simulink model "lab131"  (R2015b)
settings: Solver=ode15s  SolverMode=SingleTasking  StartTime=0.0  StopTime=0.01  RelTol=1e-3
libraries: fl_lib x8, nesl_utility x5, simulink x1
settings Model: Creator=Peter  LastModifiedBy=Peter
settings DataIOCC: LimitDataPoints=off
settings DebuggingCC: AllowSymbolicDim=on  SFUnexpectedBacktrackingDiag=error  SFNoUnconditionalDefaultTransitionDiag=error
settings ModelReferenceCC: PropagateSignalLabelsOutOfModel=on
settings GRTTargetCC: TargetLangStandard=C99 (ISO)
settings ConfigComp: CovMetricSettings=dwe  CovHtmlReporting=off  CovSaveCumulativeToWorkspaceVar=off  CovSaveSingleToWorkspaceVar=off  CovModelRefEnable=Off  CovExternalEMLEnable=on
settings ConfigurationSet: Description=Simscape Multibody

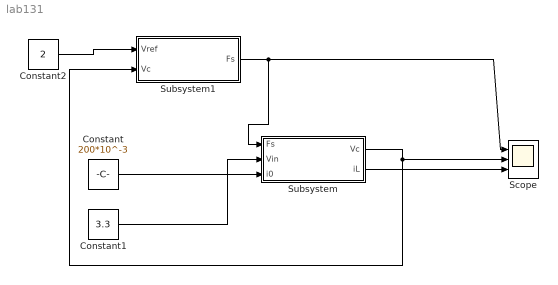
== system lab131 ==
  Constant : Constant  Value=200*10^-3
  Constant1 : Constant  Value=3.3
  Constant2 : Constant  Value=2
  Scope : Scope  NumInputPorts=3
  Subsystem : Subsystem
  Subsystem1 : Subsystem
  wires:
  Constant1/1 -> Subsystem/2(Vin)
  Subsystem/1(Vc) -> Scope/2, Subsystem1/2(Vc)
  Constant/1 -> Subsystem/3(i0)
  Subsystem1/1(Fs) -> Scope/1, Subsystem/1(Fs)
  Constant2/1 -> Subsystem1/1(Vref)
  Subsystem/2(iL) -> Scope/3

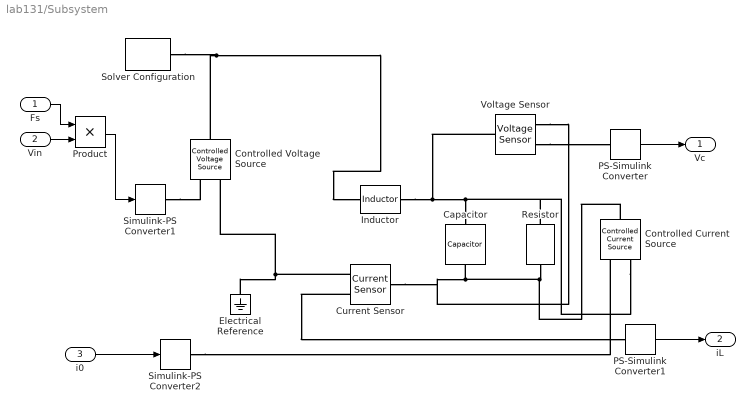
== system lab131/Subsystem ==
  Fs : Inport
  Vin : Inport  Port=2
  i0 : Inport  Port=3
  Capacitor : fl_lib/Electrical/Electrical Elements/Capacitor  c=8e-6 F  r=1e-6 Ohm  g=0 1/Ohm  i_specify=off  i_priority=None  i=0 A  i_nominal_specify=off  i_nominal_unit=A  i_nominal_value=1  v_specify=off  v_priority=None  v=0 V  v_nominal_specify=off  v_nominal_unit=V  v_nominal_value=1  vc_specify=off  vc_priority=High  vc=0 V  vc_nominal_specify=off  vc_nominal_unit=V  vc_nominal_value=1
  Controlled Current Source : fl_lib/Electrical/Electrical Sources/Controlled Current Source
  Controlled Voltage Source : fl_lib/Electrical/Electrical Sources/Controlled Voltage Source
  Current Sensor : fl_lib/Electrical/Electrical Sensors/Current Sensor
  Electrical Reference : fl_lib/Electrical/Electrical Elements/Electrical Reference
  Inductor : fl_lib/Electrical/Electrical Elements/Inductor  l=15e-6 H  r=0 Ohm  g=1e-9 1/Ohm  i_specify=off  i_priority=None  i=0 A  i_nominal_specify=off  i_nominal_unit=A  i_nominal_value=1  v_specify=off  v_priority=None  v=0 V  v_nominal_specify=off  v_nominal_unit=V  v_nominal_value=1  i_L_specify=off  i_L_priority=High  i_L=0 A  i_L_nominal_specify=off  i_L_nominal_unit=A  i_L_nominal_value=1
  PS-Simulink Converter : nesl_utility/PS-Simulink Converter  PhysicalDomain=network_engine_domain  SubClassName=ps_output  LeftPortType=input  RightPortType=output  PseudoPeriodic=off  Frequencies=[]  Unit=1  AffineConversion=off
  PS-Simulink Converter1 : nesl_utility/PS-Simulink Converter  PhysicalDomain=network_engine_domain  SubClassName=ps_output  LeftPortType=input  RightPortType=output  PseudoPeriodic=off  Frequencies=[]  Unit=1  AffineConversion=off
  Product : Product
  Resistor : fl_lib/Electrical/Electrical Elements/Resistor  R=10 Ohm  i_specify=off  i_priority=None  i=0 A  i_nominal_specify=off  i_nominal_unit=A  i_nominal_value=1  v_specify=off  v_priority=None  v=0 V  v_nominal_specify=off  v_nominal_unit=V  v_nominal_value=1
  Simulink-PS Converter1 : nesl_utility/Simulink-PS Converter  PhysicalDomain=network_engine_domain  SubClassName=ps_input  LeftPortType=input  RightPortType=output  PseudoPeriodic=off  Frequencies=[]  NoiseDistribution=none  NoiseParameters=[]  Unit=1  AffineConversion=off  FilteringAndDerivatives=provide  SimscapeFilterOrder=1  InputFilterTimeConstant=0.001  UdotUserProvided=0
  Simulink-PS Converter2 : nesl_utility/Simulink-PS Converter  PhysicalDomain=network_engine_domain  SubClassName=ps_input  LeftPortType=input  RightPortType=output  PseudoPeriodic=off  Frequencies=[]  NoiseDistribution=none  NoiseParameters=[]  Unit=1  AffineConversion=off  FilteringAndDerivatives=provide  SimscapeFilterOrder=1  InputFilterTimeConstant=0.001  UdotUserProvided=0
  Solver Configuration : nesl_utility/Solver Configuration  PhysicalDomain=network_engine_domain  SubClassName=solver  LeftPortType=input  RightPortType=generic  Accelerate=off  Tones=[]  Harmonics=[]  SimulateNoise=off  Profile=off  UseLocalSampling=off  EnableSwitchedLinearOptims=on  FrequencyDomain=off  UseCCode=off  RelTol=0.001  AbsTol=1e-06  MinStep=1e-09  ToWorkspace=off  RevertToSquareIcSolve=off  NumHomotopyIterations=100  PhasorMode=off  PhasorModeNumHarmonics=1  OverrideAbsTol=off  DoDC=off  ResidualTolerance=1e-09  UseLocalSolver=off  LocalSolverChoice=NE_BACKWARD_EULER_ADVANCER  LocalSolverSampleTime=0.001  DoFixedCost=off  MaxNonlinIter=3  MaxModeIter=2  LinearAlgebra=Sparse  DelaysMemoryBudget=1024  AutomaticFiltering=on  FilteringTimeConstant=0.001
  Voltage Sensor : fl_lib/Electrical/Electrical Sensors/Voltage Sensor
  Vc : Outport
  iL : Outport  Port=2
  wires:
  Vin/1 -> Product/2
  Fs/1 -> Product/1
  Product/1 -> Simulink-PS Converter1/1
  PS-Simulink Converter1/1 -> iL/1
  PS-Simulink Converter/1 -> Vc/1
  i0/1 -> Simulink-PS Converter2/1
  connections:
  Inductor/RConn1 -- Voltage Sensor/LConn1 -- Controlled Current Source/RConn2 -- Resistor/LConn1 -- Capacitor/LConn1
  Resistor/RConn1 -- Controlled Current Source/LConn1 -- Current Sensor/LConn1 -- Voltage Sensor/RConn2 -- Capacitor/RConn1
  Controlled Voltage Source/LConn1 -- Solver Configuration/RConn1 -- Inductor/LConn1
  Simulink-PS Converter1/RConn1 -- Controlled Voltage Source/RConn1
  Electrical Reference/LConn1 -- Current Sensor/RConn2 -- Controlled Voltage Source/RConn2
  Voltage Sensor/RConn1 -- PS-Simulink Converter/LConn1
  Current Sensor/RConn1 -- PS-Simulink Converter1/LConn1
  Simulink-PS Converter2/RConn1 -- Controlled Current Source/RConn1

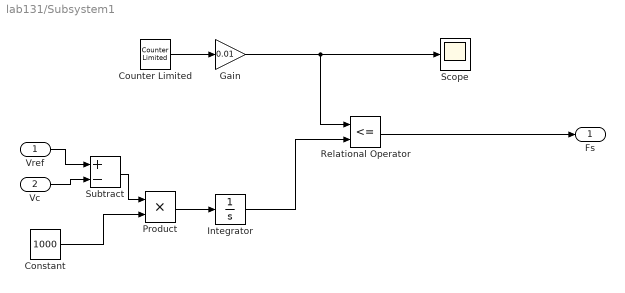
== system lab131/Subsystem1 ==
  Vref : Inport
  Vc : Inport  Port=2
  Constant : Constant  Value=1000
  Counter Limited : simulink/Sources/Counter Limited  uplimit=100  tsamp=1/100000000
  Gain : Gain  Gain=0.01
  Integrator : Integrator
  Product : Product
  Relational Operator : RelationalOperator  Operator=<=  OutDataTypeStr=boolean
  Scope : Scope
  Subtract : Sum  Inputs=+-
  Fs : Outport
  wires:
  Relational Operator/1 -> Fs/1
  Counter Limited/1 -> Gain/1
  Gain/1 -> Scope/1, Relational Operator/1
  Product/1 -> Integrator/1
  Subtract/1 -> Product/1
  Vref/1 -> Subtract/1
  Vc/1 -> Subtract/2
  Constant/1 -> Product/2
  Integrator/1 -> Relational Operator/2
